simulink model "PMSM_SquareWave"  (R2023a)
settings: Solver=VariableStepAuto  StartTime=0.0  StopTime=500e-6  MaxStep=5e-8  RelTol=1e-5
InitFcn:
  | % Loading the measurement data
  | load('MeasurementData.mat', 'PM')
libraries: fl_lib x8, SLSS x2, PMSM x2, nesl_utility x2, simulink x2
settings Model: Creator=Szalay  LastModifiedBy=Szalay
settings SolverCC: AlgebraicLoopSolver=TrustRegion
settings DebuggingCC: UnconnectedInputMsg=warning  UnconnectedOutputMsg=warning  UnconnectedLineMsg=warning
settings ModelReferenceCC: EnableRefExpFcnMdlSchedulingChecks=on
settings RTWCC: DLArmComputeVersion=19.05

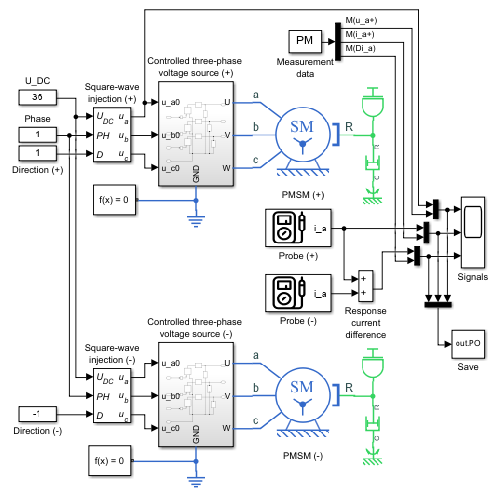
[thumbnail: Simulink's stored preview of the top-level diagram]
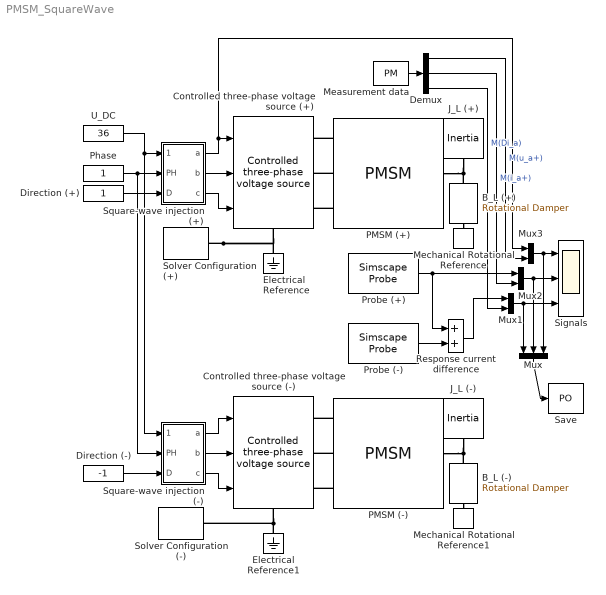
== system PMSM_SquareWave ==
  B_L (+) : fl_lib/Mechanical/Rotational Elements/Rotational Damper  D=0.001 N*m*s/rad  w_specify=off  w_priority=None  w=0 rad/s  w_nominal_specify=off  w_nominal_unit=rad/s  w_nominal_value=1  t_specify=off  t_priority=None  t=0 N*m  t_nominal_specify=off  t_nominal_unit=N*m  t_nominal_value=1
  B_L (-) : fl_lib/Mechanical/Rotational Elements/Rotational Damper  D=0.001 N*m*s/rad  w_specify=off  w_priority=None  w=0 rad/s  w_nominal_specify=off  w_nominal_unit=rad/s  w_nominal_value=1  t_specify=off  t_priority=None  t=0 N*m  t_nominal_specify=off  t_nominal_unit=N*m  t_nominal_value=1
  Controlled three-phase voltage source (+) : SLSS/Power electronics/Controlled three-phase voltage source  SystemSampleTime=-1  VariantActivationTime=update diagram  Latency=0  AutoFrameSizeCalculation=off
      settings: PortSchema="{\"entries\":[{\"content\":{\"sides\":[{\"content\":{\"connectorIds\":[\"In1\",\"In2\",\"In3\"]},\"type\":\"ConnectorPlacement.EquallySpacedRectSide\",\"uuid\":\"86f4b7c9-b4c1-4fa9-92c9-df14c018ab5a\"},{\"content\":{\"connectorIds\":[\"RConn1\",\"RConn2\",\"RConn3\"],\"side\":\"RIGHT\"},\"type\":\"ConnectorPlacement.EquallySpacedRectSide\",\"uuid\":\"262f16fa-1458-4a6c-a6cd-e957fd1dcf99\"},{\"content\":{\"side\":\"TOP\"},\"type\":\"ConnectorPlacement.EquallySpacedRectSide\",\"uuid\":\"0209afef-5535-4f88-847d-86e3dc9013d0\"},{\"content\":{\"connectorIds\":[\"RConn4\"],\"side\":\"BOTTOM\"},\"type\":\"ConnectorPlacement.EquallySpacedRectSide\",\"uuid\":\"6ee3303f-0ef7-4fac-9be7-421fc8645ecd\"}]},\"type\":\"ConnectorPlacement.EquallySpacedConnector\",\"uuid\":\"dcf2ee2c-2e64-45ce-a4a6-bf45ae3145fa\"}],\"packageUris\":[\"http://schema.mathworks.com/mf0/Connector/R2020b\"],\"version\":\"1.0\"}"
  Controlled three-phase voltage source (-) : SLSS/Power electronics/Controlled three-phase voltage source  SystemSampleTime=-1  VariantActivationTime=update diagram  Latency=0  AutoFrameSizeCalculation=off
      settings: PortSchema="{\"entries\":[{\"content\":{\"sides\":[{\"content\":{\"connectorIds\":[\"In1\",\"In2\",\"In3\"]},\"type\":\"ConnectorPlacement.EquallySpacedRectSide\",\"uuid\":\"86f4b7c9-b4c1-4fa9-92c9-df14c018ab5a\"},{\"content\":{\"connectorIds\":[\"RConn1\",\"RConn2\",\"RConn3\"],\"side\":\"RIGHT\"},\"type\":\"ConnectorPlacement.EquallySpacedRectSide\",\"uuid\":\"262f16fa-1458-4a6c-a6cd-e957fd1dcf99\"},{\"content\":{\"side\":\"TOP\"},\"type\":\"ConnectorPlacement.EquallySpacedRectSide\",\"uuid\":\"0209afef-5535-4f88-847d-86e3dc9013d0\"},{\"content\":{\"connectorIds\":[\"RConn4\"],\"side\":\"BOTTOM\"},\"type\":\"ConnectorPlacement.EquallySpacedRectSide\",\"uuid\":\"6ee3303f-0ef7-4fac-9be7-421fc8645ecd\"}]},\"type\":\"ConnectorPlacement.EquallySpacedConnector\",\"uuid\":\"dcf2ee2c-2e64-45ce-a4a6-bf45ae3145fa\"}],\"packageUris\":[\"http://schema.mathworks.com/mf0/Connector/R2020b\"],\"version\":\"1.0\"}"
  Demux : Demux  Outputs=3
  Direction (+) : Constant
  Direction (-) : Constant  Value=-1
  Electrical Reference : fl_lib/Electrical/Electrical Elements/Electrical Reference
  Electrical Reference1 : fl_lib/Electrical/Electrical Elements/Electrical Reference
  J_L (+) : fl_lib/Mechanical/Rotational Elements/Inertia  inertia=0.0001 kg*m^2  num_ports=foundation.enum.numPorts2.one  w_specify=off  w_priority=High  w=0 rad/s  w_nominal_specify=off  w_nominal_unit=rad/s  w_nominal_value=1  t_specify=off  t_priority=None  t=0 N*m  t_nominal_specify=off  t_nominal_unit=N*m  t_nominal_value=1
  J_L (-) : fl_lib/Mechanical/Rotational Elements/Inertia  inertia=0.0001 kg*m^2  num_ports=foundation.enum.numPorts2.one  w_specify=off  w_priority=High  w=0 rad/s  w_nominal_specify=off  w_nominal_unit=rad/s  w_nominal_value=1  t_specify=off  t_priority=None  t=0 N*m  t_nominal_specify=off  t_nominal_unit=N*m  t_nominal_value=1
  Measurement data : FromWorkspace  VariableName=PM  SampleTime=-1  Interpolate=off  OutputAfterFinalValue=Setting to zero
  Mechanical Rotational Reference : fl_lib/Mechanical/Rotational Elements/Mechanical Rotational Reference
  Mechanical Rotational Reference1 : fl_lib/Mechanical/Rotational Elements/Mechanical Rotational Reference
  Mux : Mux  Inputs=3
  Mux1 : Mux  Inputs=2
  Mux2 : Mux  Inputs=2
  Mux3 : Mux  Inputs=2
  PMSM (+) : PMSM/PMSM  R=0.645 Ohm  z_P=2  Psi_PM=0.02483 Wb  L_dd=145e-6 H  L_qq=188e-6 H  Gamma_0=0.16e-6 H/A  J=2e-7 kg*m^2  B=6.329e-3 N*m*s/rad  th_M0=pi/2 rad  u_a_specify=off  u_a_priority=None  u_a=0 V  u_a_nominal_specify=off  u_a_nominal_unit=V  u_a_nominal_value=1  u_b_specify=off  u_b_priority=None  u_b=0 V  u_b_nominal_specify=off  u_b_nominal_unit=V  u_b_nominal_value=1  u_c_specify=off  u_c_priority=None  u_c=0 V  u_c_nominal_specify=off  u_c_nominal_unit=V  u_c_nominal_value=1  i_a_specify=off  i_a_priority=None  i_a=0 A  i_a_nominal_specify=off  i_a_nominal_unit=A  i_a_nominal_value=1  i_b_specify=off  i_b_priority=None  i_b=0 A  i_b_nominal_specify=off  i_b_nominal_unit=A  i_b_nominal_value=1  i_c_specify=off  i_c_priority=None  i_c=0 A  i_c_nominal_specify=off  i_c_nominal_unit=A  i_c_nominal_value=1  i_n_specify=off  i_n_priority=None  i_n=0 A  i_n_nominal_specify=off  i_n_nominal_unit=A  i_n_nominal_value=1  Psi_d_specify=off  Psi_d_priority=None  Psi_d=0 Wb  Psi_d_nominal_specify=off  Psi_d_nominal_unit=Wb  Psi_d_nominal_value=1  Psi_q_specify=off  Psi_q_priority=None  Psi_q=0 Wb  Psi_q_nominal_specify=off  Psi_q_nominal_unit=Wb  Psi_q_nominal_value=1  u_d_specify=off  u_d_priority=None  u_d=0 V  u_d_nominal_specify=off  u_d_nominal_unit=V  u_d_nominal_value=1  u_q_specify=off  u_q_priority=None  u_q=0 V  u_q_nominal_specify=off  u_q_nominal_unit=V  u_q_nominal_value=1  i_d_specify=off  i_d_priority=High  i_d=0 A  i_d_nominal_specify=off  i_d_nominal_unit=A  i_d_nominal_value=1  i_q_specify=off  i_q_priority=High  i_q=0 A  i_q_nominal_specify=off  i_q_nominal_unit=A  i_q_nominal_value=1  M_E_specify=off  M_E_priority=None  M_E=0 N*m  M_E_nominal_specify=off  M_E_nominal_unit=N*m  M_E_nominal_value=1  M_L_specify=off  M_L_priority=None  M_L=0 N*m  M_L_nominal_specify=off  M_L_nominal_unit=N*m  M_L_nominal_value=1  w_M_specify=off  w_M_priority=None  w_M=0 rad/s  w_M_nominal_specify=off  w_M_nominal_unit=rad/s  w_M_nominal_value=1  w_specify=off  w_priority=None  w=0 rad/s  w_nominal_specify=off  w_nominal_unit=rad/s  w_nominal_value=1
      settings: InternalSimscapePortConfiguration="{\"Bottom\":[],\"Left\":[{\"id\":\"a\",\"label\":\"a\",\"type\":\"foundation.electrical.electrical\"},{\"id\":\"b\",\"label\":\"b\",\"type\":\"foundation.electrical.electrical\"},{\"id\":\"c\",\"label\":\"c\",\"type\":\"foundation.electrical.electrical\"}],\"Right\":[{\"id\":\"S\",\"label\":\"R\",\"type\":\"foundation.mechanical.rotational.rotational\"}],\"Top\":[]}"
  PMSM (-) : PMSM/PMSM  R=0.645 Ohm  z_P=2  Psi_PM=0.02483 Wb  L_dd=145e-6 H  L_qq=188e-6 H  Gamma_0=0.16e-6 H/A  J=2e-7 kg*m^2  B=6.329e-3 N*m*s/rad  th_M0=pi/2 rad  u_a_specify=off  u_a_priority=None  u_a=0 V  u_a_nominal_specify=off  u_a_nominal_unit=V  u_a_nominal_value=1  u_b_specify=off  u_b_priority=None  u_b=0 V  u_b_nominal_specify=off  u_b_nominal_unit=V  u_b_nominal_value=1  u_c_specify=off  u_c_priority=None  u_c=0 V  u_c_nominal_specify=off  u_c_nominal_unit=V  u_c_nominal_value=1  i_a_specify=off  i_a_priority=None  i_a=0 A  i_a_nominal_specify=off  i_a_nominal_unit=A  i_a_nominal_value=1  i_b_specify=off  i_b_priority=None  i_b=0 A  i_b_nominal_specify=off  i_b_nominal_unit=A  i_b_nominal_value=1  i_c_specify=off  i_c_priority=None  i_c=0 A  i_c_nominal_specify=off  i_c_nominal_unit=A  i_c_nominal_value=1  i_n_specify=off  i_n_priority=None  i_n=0 A  i_n_nominal_specify=off  i_n_nominal_unit=A  i_n_nominal_value=1  Psi_d_specify=off  Psi_d_priority=None  Psi_d=0 Wb  Psi_d_nominal_specify=off  Psi_d_nominal_unit=Wb  Psi_d_nominal_value=1  Psi_q_specify=off  Psi_q_priority=None  Psi_q=0 Wb  Psi_q_nominal_specify=off  Psi_q_nominal_unit=Wb  Psi_q_nominal_value=1  u_d_specify=off  u_d_priority=None  u_d=0 V  u_d_nominal_specify=off  u_d_nominal_unit=V  u_d_nominal_value=1  u_q_specify=off  u_q_priority=None  u_q=0 V  u_q_nominal_specify=off  u_q_nominal_unit=V  u_q_nominal_value=1  i_d_specify=off  i_d_priority=High  i_d=0 A  i_d_nominal_specify=off  i_d_nominal_unit=A  i_d_nominal_value=1  i_q_specify=off  i_q_priority=High  i_q=0 A  i_q_nominal_specify=off  i_q_nominal_unit=A  i_q_nominal_value=1  M_E_specify=off  M_E_priority=None  M_E=0 N*m  M_E_nominal_specify=off  M_E_nominal_unit=N*m  M_E_nominal_value=1  M_L_specify=off  M_L_priority=None  M_L=0 N*m  M_L_nominal_specify=off  M_L_nominal_unit=N*m  M_L_nominal_value=1  w_M_specify=off  w_M_priority=None  w_M=0 rad/s  w_M_nominal_specify=off  w_M_nominal_unit=rad/s  w_M_nominal_value=1  w_specify=off  w_priority=None  w=0 rad/s  w_nominal_specify=off  w_nominal_unit=rad/s  w_nominal_value=1
      settings: InternalSimscapePortConfiguration="{\"Bottom\":[],\"Left\":[{\"id\":\"a\",\"label\":\"a\",\"type\":\"foundation.electrical.electrical\"},{\"id\":\"b\",\"label\":\"b\",\"type\":\"foundation.electrical.electrical\"},{\"id\":\"c\",\"label\":\"c\",\"type\":\"foundation.electrical.electrical\"}],\"Right\":[{\"id\":\"S\",\"label\":\"R\",\"type\":\"foundation.mechanical.rotational.rotational\"}],\"Top\":[]}"
  Phase : Constant
  Probe (+) : SimscapeProbe  BoundBlock=432  Variables={i_a}
  Probe (-) : SimscapeProbe  BoundBlock=433  Variables={i_a}
  Response current difference : Sum
  Save : ToWorkspace  VariableName=PO  SampleTime=1/240000
  Signals : Scope  NumInputPorts=3
  Solver Configuration (+) : nesl_utility/Solver Configuration  PhysicalDomain=network_engine_domain  SubClassName=solver  LeftPortType=input  RightPortType=generic  Tones=[]  Harmonics=[]  SimulateNoise=off  Profile=off  UseLocalSampling=off  EnableSwitchedLinearOptims=on  FrequencyDomain=off  UseCCode=off  RelTol=0.001  AbsTol=0.001  MinStep=1e-09  ToWorkspace=off  RevertToSquareIcSolve=off  NumHomotopyIterations=100  PhasorMode=off  PhasorModeNumHarmonics=1  ConsistencySolver=NEWTON_XTOL_AFTER_FTOL  IndexReductionMethod=DerivativeReplacement  DoDC=on  ResidualTolerance=1e-09  ConsistencyTolSource=GLOBAL  ConsistencyAbsTol=0.001  ConsistencyRelTol=0.001  ConsistencyTolFactor=0.001  UseLocalSolver=off  LocalSolverChoice=NE_BACKWARD_EULER_ADVANCER  ResolveIndetEquations=on  FunctionEvalNumThread=1  LocalSolverSampleTime=0.001  DoFixedCost=off  MaxNonlinIter=3  MaxModeIter=2  ComputeImpulses=off  ImpulseIterations=2  LinearAlgebra=auto  LinearAlgebraNumThread=0  EquationFormulation=NE_TIME_EF  DelaysMemoryBudget=1024  AutomaticFiltering=on  FilteringTimeConstant=0.001  PartitionStorageMethod=AS_NEEDED  PartitionMemoryBudget=1024  PartitionMethod=ROBUST
  Solver Configuration (-) : nesl_utility/Solver Configuration  PhysicalDomain=network_engine_domain  SubClassName=solver  LeftPortType=input  RightPortType=generic  Tones=[]  Harmonics=[]  SimulateNoise=off  Profile=off  UseLocalSampling=off  EnableSwitchedLinearOptims=on  FrequencyDomain=off  UseCCode=off  RelTol=0.001  AbsTol=0.001  MinStep=1e-09  ToWorkspace=off  RevertToSquareIcSolve=off  NumHomotopyIterations=100  PhasorMode=off  PhasorModeNumHarmonics=1  ConsistencySolver=NEWTON_XTOL_AFTER_FTOL  IndexReductionMethod=DerivativeReplacement  DoDC=on  ResidualTolerance=1e-09  ConsistencyTolSource=GLOBAL  ConsistencyAbsTol=0.001  ConsistencyRelTol=0.001  ConsistencyTolFactor=0.001  UseLocalSolver=off  LocalSolverChoice=NE_BACKWARD_EULER_ADVANCER  ResolveIndetEquations=on  FunctionEvalNumThread=1  LocalSolverSampleTime=0.001  DoFixedCost=off  MaxNonlinIter=3  MaxModeIter=2  ComputeImpulses=off  ImpulseIterations=2  LinearAlgebra=auto  LinearAlgebraNumThread=0  EquationFormulation=NE_TIME_EF  DelaysMemoryBudget=1024  AutomaticFiltering=on  FilteringTimeConstant=0.001  PartitionStorageMethod=AS_NEEDED  PartitionMemoryBudget=1024  PartitionMethod=ROBUST
  Square-wave injection (+) : Subsystem
      mask Display:
      | port_label('input', 1, '\itU_{DC}', 'texmode', 'on');
      | port_label('input', 2, '\itPH', 'texmode', 'on');
      | port_label('input', 3, '\itD', 'texmode', 'on');
      | 
      | port_label('output', 1, '\itu_a', 'texmode', 'on');
      | port_label('output', 2, '\itu_b', 'texmode', 'on');
      | port_label('output', 3, '\itu_c', 'texmode', 'on');
  Square-wave injection (-) : Subsystem
      mask Display:
      | port_label('input', 1, '\itU_{DC}', 'texmode', 'on');
      | port_label('input', 2, '\itPH', 'texmode', 'on');
      | port_label('input', 3, '\itD', 'texmode', 'on');
      | 
      | port_label('output', 1, '\itu_a', 'texmode', 'on');
      | port_label('output', 2, '\itu_b', 'texmode', 'on');
      | port_label('output', 3, '\itu_c', 'texmode', 'on');
  U_DC : Constant  Value=36
  wires:
  Measurement data/1 -> Demux/1
  Demux/3 -> Mux1/2  "M(Di_a)"
  Demux/2 -> Mux2/2  "M(i_a+)"
  Demux/1 -> Mux3/2  "M(u_a+)"
  Response current difference/1 -> Mux1/1
  Direction (+)/1 -> Square-wave injection (+)/3(D)
  Probe (+)/1 -> Response current difference/1, Mux2/1
  Direction (-)/1 -> Square-wave injection (-)/3(D)
  Phase/1 -> Square-wave injection (+)/2(PH), Square-wave injection (-)/2(PH)
  U_DC/1 -> Square-wave injection (+)/1(U_DC), Square-wave injection (-)/1(U_DC)
  Probe (-)/1 -> Response current difference/2
  Mux/1 -> Save/1
  Mux2/1 -> Mux/2, Signals/2
  Mux1/1 -> Mux/1, Signals/3
  Mux3/1 -> Mux/3, Signals/1
  Square-wave injection (+)/1(a) -> Mux3/1, Controlled three-phase voltage source (+)/1
  Square-wave injection (+)/3(c) -> Controlled three-phase voltage source (+)/3
  Square-wave injection (+)/2(b) -> Controlled three-phase voltage source (+)/2
  Square-wave injection (-)/2(b) -> Controlled three-phase voltage source (-)/2
  Square-wave injection (-)/3(c) -> Controlled three-phase voltage source (-)/3
  Square-wave injection (-)/1(a) -> Controlled three-phase voltage source (-)/1
  connections:
  B_L (+)/LConn1 -- PMSM (+)/RConn1 -- J_L (+)/LConn1
  Solver Configuration (+)/RConn1 -- Controlled three-phase voltage source (+)/RConn4 -- Electrical Reference/LConn1
  B_L (+)/RConn1 -- Mechanical Rotational Reference/LConn1
  B_L (-)/LConn1 -- PMSM (-)/RConn1 -- J_L (-)/LConn1
  Electrical Reference1/LConn1 -- Controlled three-phase voltage source (-)/RConn4 -- Solver Configuration (-)/RConn1
  B_L (-)/RConn1 -- Mechanical Rotational Reference1/LConn1
  PMSM (+)/LConn1 -- Controlled three-phase voltage source (+)/RConn1
  PMSM (+)/LConn2 -- Controlled three-phase voltage source (+)/RConn2
  PMSM (+)/LConn3 -- Controlled three-phase voltage source (+)/RConn3
  PMSM (-)/LConn1 -- Controlled three-phase voltage source (-)/RConn1
  PMSM (-)/LConn2 -- Controlled three-phase voltage source (-)/RConn2
  PMSM (-)/LConn3 -- Controlled three-phase voltage source (-)/RConn3

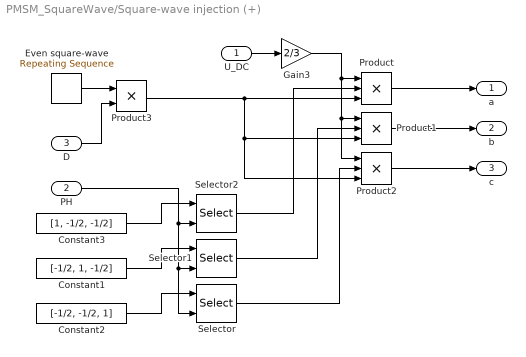
== system PMSM_SquareWave/Square-wave injection (+) ==
  U_DC : Inport
  PH : Inport  Port=2
  D : Inport  Port=3
  Constant1 : Constant  Value=[-1/2, 1, -1/2]
  Constant2 : Constant  Value=[-1/2, -1/2, 1]
  Constant3 : Constant  Value=[1, -1/2, -1/2]
  Even square-wave : simulink/Sources/Repeating Sequence  rep_seq_t=[0 1 1.05 2 2.05 4 4.05 5 5.05 2500]*75e-6  rep_seq_y="[0 0 1     1 -1    -1 1     1 0     0]"
  Gain3 : Gain  Gain=2/3
  Product : Product  Inputs=3
  Product1 : Product  Inputs=3
  Product2 : Product  Inputs=3
  Product3 : Product
  Selector : Selector  InputPortWidth=3  IndexOptions=Index vector (port)  Indices=[1 3]  OutputSizes=1
  Selector1 : Selector  InputPortWidth=3  IndexOptions=Index vector (port)  Indices=[1 3]  OutputSizes=1
  Selector2 : Selector  InputPortWidth=3  IndexOptions=Index vector (port)  Indices=[1 3]  OutputSizes=1
  a : Outport
  b : Outport  Port=2
  c : Outport  Port=3
  wires:
  Gain3/1 -> Product/1, Product2/1, Product1/1
  Even square-wave/1 -> Product3/1
  D/1 -> Product3/2
  U_DC/1 -> Gain3/1
  Product1/1 -> b/1
  Product2/1 -> c/1
  Product/1 -> a/1
  Product3/1 -> Product2/3, Product1/3, Product/3
  Selector2/1 -> Product/2
  Selector1/1 -> Product1/2
  Selector/1 -> Product2/2
  Constant3/1 -> Selector2/1
  Constant1/1 -> Selector1/1
  Constant2/1 -> Selector/1
  PH/1 -> Selector2/2, Selector1/2, Selector/2

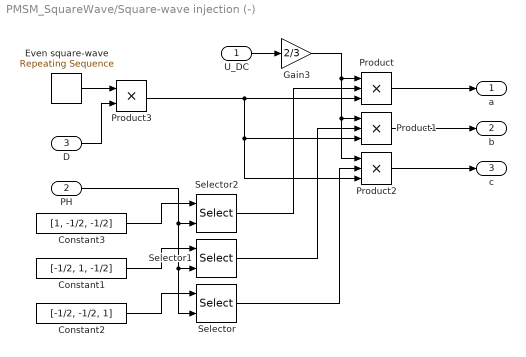
== system PMSM_SquareWave/Square-wave injection (-) ==
  U_DC : Inport
  PH : Inport  Port=2
  D : Inport  Port=3
  Constant1 : Constant  Value=[-1/2, 1, -1/2]
  Constant2 : Constant  Value=[-1/2, -1/2, 1]
  Constant3 : Constant  Value=[1, -1/2, -1/2]
  Even square-wave : simulink/Sources/Repeating Sequence  rep_seq_t=[0 1 1.05 2 2.05 4 4.05 5 5.05 2500]*75e-6  rep_seq_y="[0 0 1     1 -1    -1 1     1 0     0]"
  Gain3 : Gain  Gain=2/3
  Product : Product  Inputs=3
  Product1 : Product  Inputs=3
  Product2 : Product  Inputs=3
  Product3 : Product
  Selector : Selector  InputPortWidth=3  IndexOptions=Index vector (port)  Indices=[1 3]  OutputSizes=1
  Selector1 : Selector  InputPortWidth=3  IndexOptions=Index vector (port)  Indices=[1 3]  OutputSizes=1
  Selector2 : Selector  InputPortWidth=3  IndexOptions=Index vector (port)  Indices=[1 3]  OutputSizes=1
  a : Outport
  b : Outport  Port=2
  c : Outport  Port=3
  wires:
  PH/1 -> Selector/2, Selector1/2, Selector2/2
  Constant2/1 -> Selector/1
  Constant1/1 -> Selector1/1
  Constant3/1 -> Selector2/1
  Selector/1 -> Product2/2
  Selector1/1 -> Product1/2
  Selector2/1 -> Product/2
  Product3/1 -> Product/3, Product1/3, Product2/3
  Product/1 -> a/1
  Product2/1 -> c/1
  Product1/1 -> b/1
  U_DC/1 -> Gain3/1
  D/1 -> Product3/2
  Even square-wave/1 -> Product3/1
  Gain3/1 -> Product1/1, Product2/1, Product/1
